simulink model "estimate_1"  (R2020b)
settings: Solver=VariableStepAuto  StartTime=0.0  StopTime=29.995  RelTol=1e-3
undefined symbols (not defined in the file or in its folder): A_kalman, L
settings Model: Creator=renato  LastModifiedBy=renato

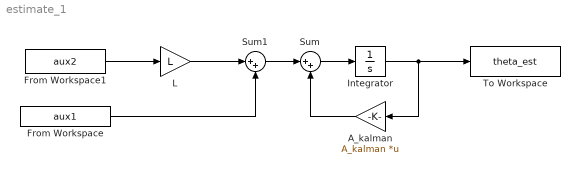
== system estimate_1 ==
  A_kalman : Gain  Gain=A_kalman  Multiplication=Matrix(K*u)
  From Workspace : FromWorkspace  VariableName=aux1
  From Workspace1 : FromWorkspace  VariableName=aux2
  Integrator : Integrator
  L : Gain  Gain=L
  Sum : Sum  Inputs=|++
  Sum1 : Sum  Inputs=|++
  To Workspace : ToWorkspace  VariableName=theta_est  SampleTime=0.005
  wires:
  Integrator/1 -> To Workspace/1, A_kalman/1
  Sum/1 -> Integrator/1
  A_kalman/1 -> Sum/2
  Sum1/1 -> Sum/1
  L/1 -> Sum1/1
  From Workspace/1 -> Sum1/2
  From Workspace1/1 -> L/1
